simulink model "fourCars"  (R2024a)
settings: Solver=FixedStepAuto  StartTime=0.0  StopTime=config.t_max  FixedStep=config.timestep  RelTol=1e-3
undefined symbols (not defined in the file or in its folder): agentsInfo, config, DiscIntNeverNeededParam, Sim3dSensor
libraries: sim3dlib x6, dspvision x1, visionsinks x1
settings Model: Creator=alexs  LastModifiedBy=alexs

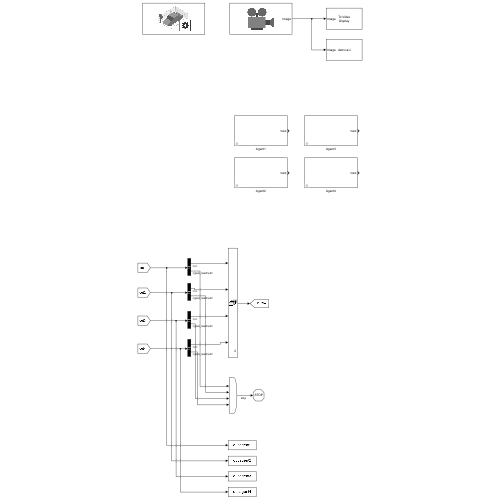
[thumbnail: Simulink's stored preview of the top-level diagram]
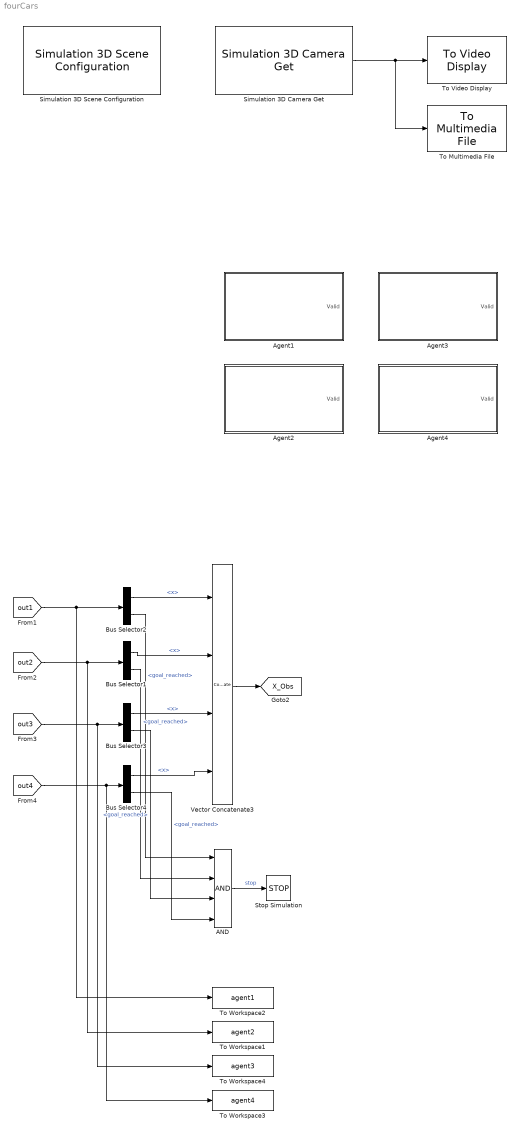
== system fourCars ==
  AND : Logic  Inputs=4  IconShape=distinctive  AllPortsSameDT=off  OutDataTypeStr=boolean
  Agent1 : Subsystem  mask{id=1, allAgentsInfo=agentsInfo}
      mask prompts: id "Identifier"; allAgentsInfo "Agents information"
  Agent2 : Subsystem  mask{id=2, allAgentsInfo=agentsInfo}
      mask prompts: id "Identifier"; allAgentsInfo "Agents information"
  Agent3 : Subsystem  mask{id=3, allAgentsInfo=agentsInfo}
      mask prompts: id "Identifier"; allAgentsInfo "Agents information"
  Agent4 : Subsystem  mask{id=4, allAgentsInfo=agentsInfo}
      mask prompts: id "Identifier"; allAgentsInfo "Agents information"
  Bus Selector{1..4} (4 alike) : BusSelector  OutputSignals=x,goal_reached
  Simulation 3D Camera Get : sim3dlib/Simulation 3D Camera Get  Priority=1  sensorTag=Sim3dSensor�  sensorId=1  sensorName=Sim3dSensor�  vehTagList={'Scene Origin';'actor1000'}  vehTag=Scene Origin  mountLoc=Origin  offsetFlag=on  tmountOffset=cameraTranslation  rmountOffset=cameraRotation  HorizontalResolution=1280  VerticalResolution=720  HorizontalFOV=60  SampleTime=-1  mountPoint=[0 0 40]  mountOrientation=[0 -90 -90]  aMode=5  ID=1
      settings: LibrarySourceBlock=sl3dlib/Simulation 3D/Utilities/Simulation 3D Camera Get
  Simulation 3D Scene Configuration : sim3dlib/Simulation 3D Scene Configuration  Priority=0  ProjectFormat=Default Scenes  SceneDesc=Empty scene  ProjectName=C:\Program Files\MATLAB\R2024a\toolbox\shared\sim3d_projects\automotive_project_windows\UE\WindowsNoEditor\VehicleSimulation.exe  ScenePath=/Game/Maps/HwStrght  EnableOpenDRIVE=off  vehTagList={'Custom';'Scene Origin';'actor1000'}  vehTag=Scene Origin  FreeCameraInitialTranslation=[0, 0, 0]  FreeCameraDefaultInitialTranslation=[-6, 0, 2]  FreeCameraInitialRotation=[0, 0, 0]  FreeCameraDefaultInitialRotation=[0, -15, 0]  OpVisEn=off  Ts=config.timestep  EnableWindow=off  EnableRemoteAccess=off  EnableWeather=off  SunAzimuth=90  SunAltitude=40.0  EnableGeospatialSun=off  Latitude=0  Longitude=0  Date=2023-01-01  Time=10:30:00  GeoTimeZone=-5.0  SunDaylightSaving=off  wind=1  clouds=10  EnableVolumetricClouds=off  CloudCoverage=0  CloudAltitude=6  fog=0  rain=0  RaindropsEffect=off  SnowDensity=0  EnableGeospatial=off  UseTrueOrigin=off  OriginHeight=200  OriginLatitude=40.744652  OriginLongitude=-73.988864  MapStyle=Aerial  AdditionalAssetIDs=[]  UseAdvancedSunSky=off  SolarTime=11  TimeZone=-5  Day=21  Month=9  Year=2022  UseDaylightSavingTime=on  DSTStartDay=10  DSTStartMonth=3  DSTEndDay=3  DSTEndMonth=11  DSTSwitchHour=2  sensorTag=MainCamera1  sensorId=1  sensorName=MainCamera1  mountLoc=Origin  offsetFlag=off  tmountOffset=[0, 0, 0]  rmountOffset=[0, 0, 0]  HorizontalResolution=1280  VerticalResolution=720  HorizontalFOV=60  mountPoint=[0 0 0]  mountOrientation=[0 0 0]  aMode=5  ID=1  GeoTrigger=Inactive
      settings: LibrarySourceBlock=sl3dlib/Simulation 3D/Environment/Simulation 3D Scene Configuration
  Stop Simulation : Stop
  To Multimedia File : dspvision/To Multimedia File  outputFilename=demo.avi  streamSelection=Video only  videoCompressor=None (uncompressed)  audioCompressor=None (uncompressed)  imagePorts=One multidimensional signal  fileType=AVI  audioDatatype=Determine from input data type  fourcc=RGB  audioBitRate=128  audioQuality=75  videoQuality=75  mj2000CompFactor=10
      settings: LibrarySourceBlock=visionsinks/To Multimedia File
  To Video Display : visionsinks/To Video Display  windowSizeMode=Normal  openAtMdlStart=on  fullScreen=off  videoWindowX=536805376  videoWindowY=536805376  saveWindowSize=off  videoWindowWidth=808  videoWindowHeight=639  inputColorFormat=RGB  inputType=Obsolete  imagePorts=One multidimensional signal  OutputDevice=On-screen video monitor  dataOrg=Column-major  isWindowOpen=off
  To Workspace1 : ToWorkspace  VariableName=agent2  SaveFormat=Timeseries  SampleTime=-1
  To Workspace2 : ToWorkspace  VariableName=agent1  SaveFormat=Timeseries  SampleTime=-1
  To Workspace3 : ToWorkspace  VariableName=agent4  SaveFormat=Timeseries  SampleTime=-1
  To Workspace4 : ToWorkspace  VariableName=agent3  SaveFormat=Timeseries  SampleTime=-1
  Vector Concatenate3 : Concatenate  NumInputs=4  Mode=Multidimensional array  ConcatenateDimension=2
  tag scope: X_Obs=global
  wires:
  Simulation 3D Camera Get/1 -> To Multimedia File/1, To Video Display/1
  [out1] -> To Workspace2/1, Bus Selector2/1
  Bus Selector2/1 -> Vector Concatenate3/1  "<x>"
  Vector Concatenate3/1 -> [X_Obs]
  Bus Selector2/2 -> AND/1  "<goal_reached>"
  AND/1 -> Stop Simulation/1  "stop"
  [out2] -> Bus Selector1/1, To Workspace1/1
  Bus Selector1/1 -> Vector Concatenate3/2  "<x>"
  Bus Selector1/2 -> AND/2  "<goal_reached>"
  [out3] -> To Workspace4/1, Bus Selector3/1
  [out4] -> To Workspace3/1, Bus Selector4/1
  Bus Selector3/1 -> Vector Concatenate3/3  "<x>"
  Bus Selector4/1 -> Vector Concatenate3/4  "<x>"
  Bus Selector3/2 -> AND/3  "<goal_reached>"
  Bus Selector4/2 -> AND/4  "<goal_reached>"

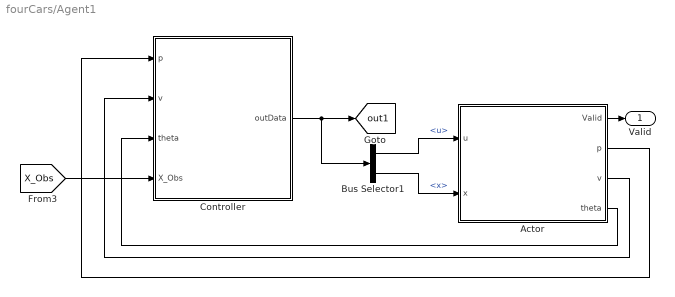
== system fourCars/Agent1 ==
  Actor : Subsystem
  Bus Selector1 : BusSelector  OutputSignals=u,x
  Controller : Subsystem  mask{id=id, allAgentsInfo=agentsInfo}
      mask prompts: id "Identifier"; allAgentsInfo "Information for all agents"
  Valid : Outport
  tag scope: out1=global
  wires:
  Actor/3(v) -> Controller/2(v)
  Controller/1(outData) -> Bus Selector1/1, [out1]
  Actor/2(p) -> Controller/1(p)
  Bus Selector1/1 -> Actor/1(u)  "<u>"
  [X_Obs] -> Controller/4(X_Obs)
  Actor/1(Valid) -> Valid/1
  Actor/4(theta) -> Controller/3(theta)
  Bus Selector1/2 -> Actor/2(x)  "<x>"

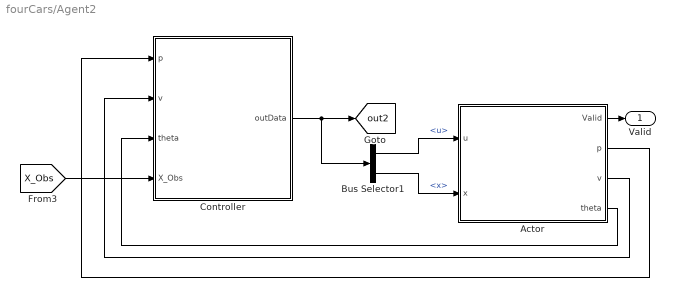
== system fourCars/Agent2 ==
  Actor : Subsystem
  Bus Selector1 : BusSelector  OutputSignals=u,x
  Controller : Subsystem  mask{id=id, allAgentsInfo=agentsInfo}
      mask prompts: id "Identifier"; allAgentsInfo "Information for all agents"
  Valid : Outport
  tag scope: out2=global
  wires:
  Bus Selector1/2 -> Actor/2(x)  "<x>"
  Actor/4(theta) -> Controller/3(theta)
  Actor/1(Valid) -> Valid/1
  [X_Obs] -> Controller/4(X_Obs)
  Bus Selector1/1 -> Actor/1(u)  "<u>"
  Actor/2(p) -> Controller/1(p)
  Controller/1(outData) -> [out2], Bus Selector1/1
  Actor/3(v) -> Controller/2(v)

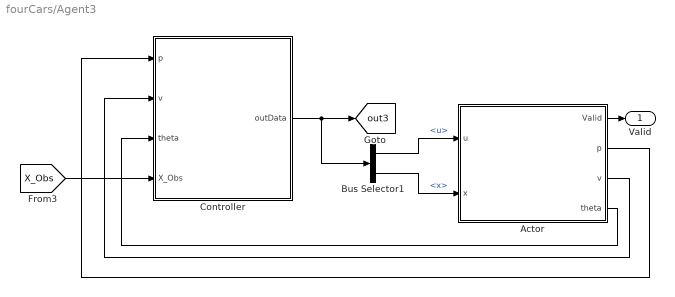
== system fourCars/Agent3 ==
  Actor : Subsystem
  Bus Selector1 : BusSelector  OutputSignals=u,x
  Controller : Subsystem  mask{id=id, allAgentsInfo=agentsInfo}
      mask prompts: id "Identifier"; allAgentsInfo "Information for all agents"
  Valid : Outport
  tag scope: out3=global
  wires:
  Bus Selector1/2 -> Actor/2(x)  "<x>"
  Actor/4(theta) -> Controller/3(theta)
  Actor/1(Valid) -> Valid/1
  [X_Obs] -> Controller/4(X_Obs)
  Bus Selector1/1 -> Actor/1(u)  "<u>"
  Actor/2(p) -> Controller/1(p)
  Controller/1(outData) -> [out3], Bus Selector1/1
  Actor/3(v) -> Controller/2(v)

== system fourCars/Agent4 ==
  Actor : Subsystem
  Bus Selector1 : BusSelector  OutputSignals=u,x
  Controller : Subsystem  mask{id=id, allAgentsInfo=agentsInfo}
      mask prompts: id "Identifier"; allAgentsInfo "Information for all agents"
  Valid : Outport
  tag scope: out4=global
  wires:
  Actor/3(v) -> Controller/2(v)
  Controller/1(outData) -> Bus Selector1/1, [out4]
  Actor/2(p) -> Controller/1(p)
  Bus Selector1/1 -> Actor/1(u)  "<u>"
  [X_Obs] -> Controller/4(X_Obs)
  Actor/1(Valid) -> Valid/1
  Actor/4(theta) -> Controller/3(theta)
  Bus Selector1/2 -> Actor/2(x)  "<x>"

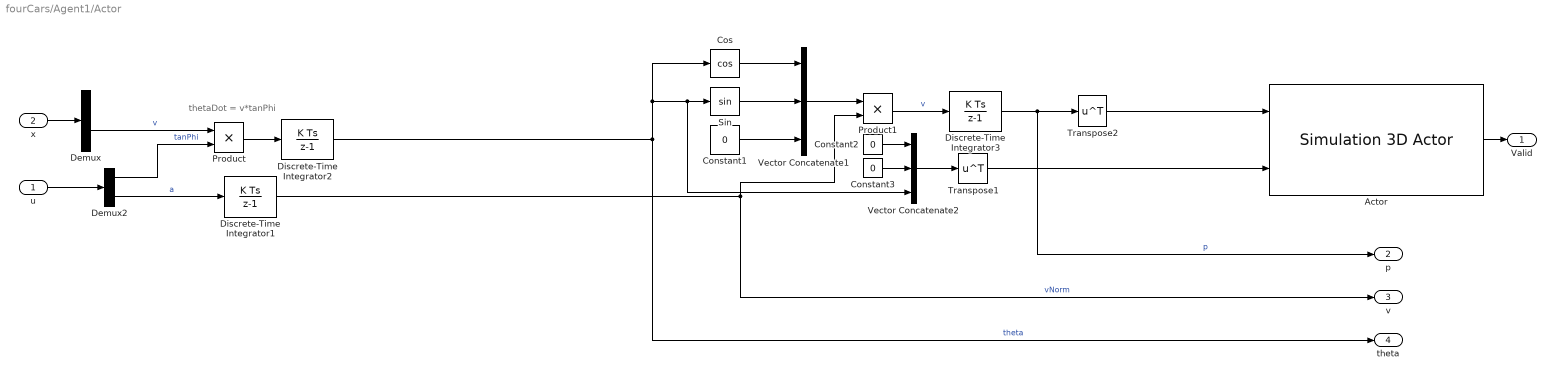
== system fourCars/Agent1/Actor ==
  note: thetaDot = v*tanPhi
  u : Inport
  x : Inport  Port=2
  Actor : sim3dlib/Simulation 3D Actor  Priority=1  ActorName=actor1  ParentName=Scene Origin  Operation=Create at setup  InitScriptText=|  SampleTime=-1  Translation=agentsInfo{id}.p'  Rotation=single([0 0 0])  Scale=single([1 1 1])  InputsText=actor1.Translation actor1.Rotation  aMode=5  ActorTag=actor1  ActorType=Sim3dActor  ID=C
      | % Reserved keywords:
      | % - Actor : handle to this actor object
      | % - World : handle to the world object
      | 
      | % Examples:
      | 
      | % Create a primitive geometry (optional)
      | 
      | % Actor.createShape('sphere', [allAgentsInfo{id}.shape(1) allAgentsInfo{id}.shape(2) 1]);
      | 
      | 
      | % Initialize values (optional)
      | % Actor.Scale = 1;
      | % Actor.Gravity = false;
      | % Actor.Physics = true;
      | % Actor.Color = [0 0 1];
      | % Actor.Shininess = 0;
      | % Actor.Mobility = sim3d.utils.MobilityTypes.Movable;
      | % Actor.Shadows = false;
  Constant1 : Constant  Value=0
  Constant2 : Constant  Value=0
  Constant3 : Constant  Value=0
  Cos : Trigonometry  Operator=cos
  Demux : Demux  Outputs=5
  Demux2 : Demux  Outputs=2
  Discrete-Time Integrator1 : DiscreteIntegrator  InitialCondition=agentsInfo{id}.v  SampleTime=-1  LimitOutput=on  UpperSaturationLimit=config.v_max/sqrt(2)  LowerSaturationLimit=-config.v_max/sqrt(2)  ICPrevOutput=DiscIntNeverNeededParam  ICPrevScaledInput=DiscIntNeverNeededParam
  Discrete-Time Integrator2 : DiscreteIntegrator  InitialCondition=agentsInfo{id}.theta  SampleTime=-1  ICPrevOutput=DiscIntNeverNeededParam  ICPrevScaledInput=DiscIntNeverNeededParam
  Discrete-Time Integrator3 : DiscreteIntegrator  InitialCondition=agentsInfo{id}.p  SampleTime=-1  UpperSaturationLimit=config.vMax  LowerSaturationLimit=-config.vMax  ICPrevOutput=DiscIntNeverNeededParam  ICPrevScaledInput=DiscIntNeverNeededParam
  Product : Product
  Product1 : Product
  Sin : Trigonometry
  Transpose1 : Math  Operator=transpose
  Transpose2 : Math  Operator=transpose
  Vector Concatenate1 : Concatenate  NumInputs=3
  Vector Concatenate2 : Concatenate  NumInputs=3
  Valid : Outport
  p : Outport  Port=2
  v : Outport  Port=3
  theta : Outport  Port=4
  wires:
  Actor/1 -> Valid/1
  Product/1 -> Discrete-Time Integrator2/1
  Demux2/1 -> Product/2  "tanPhi"
  Demux2/2 -> Discrete-Time Integrator1/1  "a"
  Discrete-Time Integrator2/1 -> Vector Concatenate2/3, Sin/1, Cos/1, theta/1  "theta"
  u/1 -> Demux2/1
  Discrete-Time Integrator1/1 -> Product1/2, v/1  "vNorm"
  Cos/1 -> Vector Concatenate1/1
  Sin/1 -> Vector Concatenate1/2
  Constant1/1 -> Vector Concatenate1/3
  Vector Concatenate1/1 -> Product1/1
  Product1/1 -> Discrete-Time Integrator3/1  "v"
  Discrete-Time Integrator3/1 -> p/1, Transpose2/1  "p"
  Transpose2/1 -> Actor/1
  x/1 -> Demux/1
  Demux/4 -> Product/1  "v"
  Constant2/1 -> Vector Concatenate2/1
  Constant3/1 -> Vector Concatenate2/2
  Vector Concatenate2/1 -> Transpose1/1
  Transpose1/1 -> Actor/2

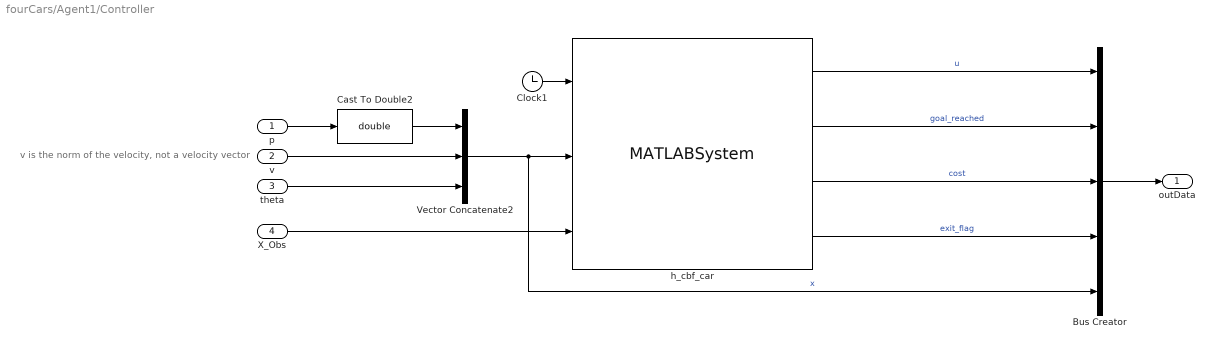
== system fourCars/Agent1/Controller ==
  note: v is the norm of the velocity, not a velocity vector
  p : Inport
  v : Inport  Port=2
  theta : Inport  Port=3
  X_Obs : Inport  Port=4
  Bus Creator : BusCreator  Inputs=5
  Cast To Double2 : DataTypeConversion  OutDataTypeStr=double  SaturateOnIntegerOverflow=off  RndMeth=Floor
  Clock1 : Clock
  Vector Concatenate2 : Concatenate  NumInputs=3
  h_cbf_car : MATLABSystem  System=h_cbf_car  id=id  config=config  agents_info=agentsInfo  SimulateUsing=Interpreted execution
      mask Type: h_cbf_car
      mask Display:
      | disp('h_cbf_car');
      | port_label('input',1,'t');
      | port_label('input',2,'x');
      | port_label('input',3,'X_obs');
      | port_label('output',1,'u');
      | port_label('output',2,'goal_reached');
      | port_label('output',3,'cost');
      | port_label('output',4,'exit_flag');
  outData : Outport
  wires:
  Vector Concatenate2/1 -> Bus Creator/5, h_cbf_car/2  "x"
  h_cbf_car/4 -> Bus Creator/4  "exit_flag"
  Bus Creator/1 -> outData/1
  Clock1/1 -> h_cbf_car/1
  h_cbf_car/3 -> Bus Creator/3  "cost"
  Cast To Double2/1 -> Vector Concatenate2/1
  h_cbf_car/1 -> Bus Creator/1  "u"
  p/1 -> Cast To Double2/1
  X_Obs/1 -> h_cbf_car/3
  h_cbf_car/2 -> Bus Creator/2  "goal_reached"
  v/1 -> Vector Concatenate2/2
  theta/1 -> Vector Concatenate2/3

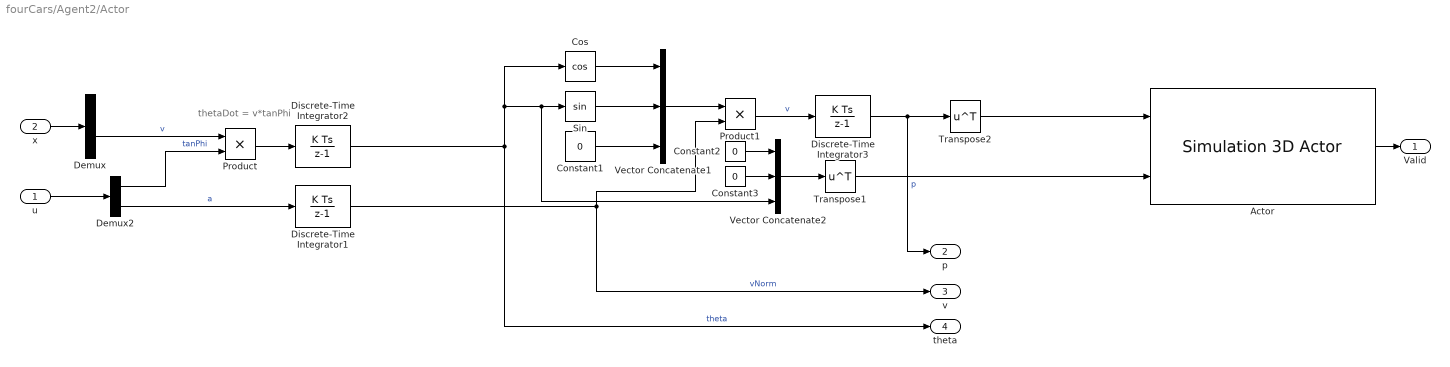
== system fourCars/Agent2/Actor ==
  note: thetaDot = v*tanPhi
  u : Inport
  x : Inport  Port=2
  Actor : sim3dlib/Simulation 3D Actor  Priority=1  ActorName=actor2  ParentName=Scene Origin  Operation=Create at setup  InitScriptText=|  SampleTime=-1  Translation=agentsInfo{id}.p'  Rotation=single([0 0 0])  Scale=single([1 1 1])  InputsText=actor2.Translation actor2.Rotation  aMode=5  ActorTag=actor2  ActorType=Sim3dActor  ID=C
      | % Reserved keywords:
      | % - Actor : handle to this actor object
      | % - World : handle to the world object
      | 
      | % Examples:
      | 
      | % Create a primitive geometry (optional)
      | 
      | % Actor.createShape('sphere', [allAgentsInfo{id}.shape(1) allAgentsInfo{id}.shape(2) 1]);
      | 
      | 
      | % Initialize values (optional)
      | % Actor.Scale = 1;
      | % Actor.Gravity = false;
      | % Actor.Physics = true;
      | % Actor.Color = [0 0 1];
      | % Actor.Shininess = 0;
      | % Actor.Mobility = sim3d.utils.MobilityTypes.Movable;
      | % Actor.Shadows = false;
  Constant1 : Constant  Value=0
  Constant2 : Constant  Value=0
  Constant3 : Constant  Value=0
  Cos : Trigonometry  Operator=cos
  Demux : Demux  Outputs=5
  Demux2 : Demux  Outputs=2
  Discrete-Time Integrator1 : DiscreteIntegrator  InitialCondition=agentsInfo{id}.v  SampleTime=-1  LimitOutput=on  UpperSaturationLimit=config.v_max/sqrt(2)  LowerSaturationLimit=-config.v_max/sqrt(2)  ICPrevOutput=DiscIntNeverNeededParam  ICPrevScaledInput=DiscIntNeverNeededParam
  Discrete-Time Integrator2 : DiscreteIntegrator  InitialCondition=agentsInfo{id}.theta  SampleTime=-1  ICPrevOutput=DiscIntNeverNeededParam  ICPrevScaledInput=DiscIntNeverNeededParam
  Discrete-Time Integrator3 : DiscreteIntegrator  InitialCondition=agentsInfo{id}.p  SampleTime=-1  UpperSaturationLimit=config.vMax  LowerSaturationLimit=-config.vMax  ICPrevOutput=DiscIntNeverNeededParam  ICPrevScaledInput=DiscIntNeverNeededParam
  Product : Product
  Product1 : Product
  Sin : Trigonometry
  Transpose1 : Math  Operator=transpose
  Transpose2 : Math  Operator=transpose
  Vector Concatenate1 : Concatenate  NumInputs=3
  Vector Concatenate2 : Concatenate  NumInputs=3
  Valid : Outport
  p : Outport  Port=2
  v : Outport  Port=3
  theta : Outport  Port=4
  wires:
  Transpose1/1 -> Actor/2
  Vector Concatenate2/1 -> Transpose1/1
  Constant3/1 -> Vector Concatenate2/2
  Constant2/1 -> Vector Concatenate2/1
  Demux/4 -> Product/1  "v"
  x/1 -> Demux/1
  Transpose2/1 -> Actor/1
  Discrete-Time Integrator3/1 -> Transpose2/1, p/1  "p"
  Product1/1 -> Discrete-Time Integrator3/1  "v"
  Vector Concatenate1/1 -> Product1/1
  Constant1/1 -> Vector Concatenate1/3
  Sin/1 -> Vector Concatenate1/2
  Cos/1 -> Vector Concatenate1/1
  Discrete-Time Integrator1/1 -> v/1, Product1/2  "vNorm"
  u/1 -> Demux2/1
  Discrete-Time Integrator2/1 -> theta/1, Cos/1, Sin/1, Vector Concatenate2/3  "theta"
  Demux2/2 -> Discrete-Time Integrator1/1  "a"
  Demux2/1 -> Product/2  "tanPhi"
  Product/1 -> Discrete-Time Integrator2/1
  Actor/1 -> Valid/1

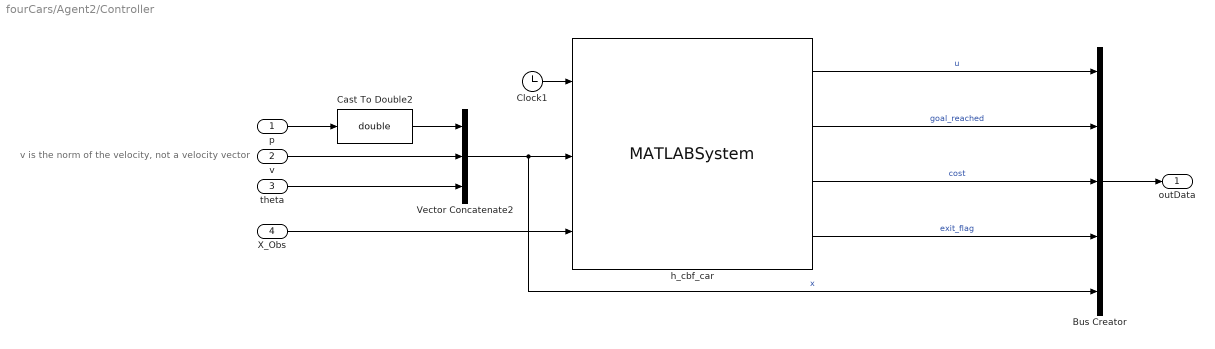
== system fourCars/Agent2/Controller ==
  note: v is the norm of the velocity, not a velocity vector
  p : Inport
  v : Inport  Port=2
  theta : Inport  Port=3
  X_Obs : Inport  Port=4
  Bus Creator : BusCreator  Inputs=5
  Cast To Double2 : DataTypeConversion  OutDataTypeStr=double  SaturateOnIntegerOverflow=off  RndMeth=Floor
  Clock1 : Clock
  Vector Concatenate2 : Concatenate  NumInputs=3
  h_cbf_car : MATLABSystem  System=h_cbf_car  id=id  config=config  agents_info=agentsInfo  SimulateUsing=Interpreted execution
      mask Type: h_cbf_car
      mask Display:
      | disp('h_cbf_car');
      | port_label('input',1,'t');
      | port_label('input',2,'x');
      | port_label('input',3,'X_obs');
      | port_label('output',1,'u');
      | port_label('output',2,'goal_reached');
      | port_label('output',3,'cost');
      | port_label('output',4,'exit_flag');
  outData : Outport
  wires:
  theta/1 -> Vector Concatenate2/3
  v/1 -> Vector Concatenate2/2
  h_cbf_car/2 -> Bus Creator/2  "goal_reached"
  X_Obs/1 -> h_cbf_car/3
  p/1 -> Cast To Double2/1
  h_cbf_car/1 -> Bus Creator/1  "u"
  Cast To Double2/1 -> Vector Concatenate2/1
  h_cbf_car/3 -> Bus Creator/3  "cost"
  Clock1/1 -> h_cbf_car/1
  Bus Creator/1 -> outData/1
  h_cbf_car/4 -> Bus Creator/4  "exit_flag"
  Vector Concatenate2/1 -> h_cbf_car/2, Bus Creator/5  "x"

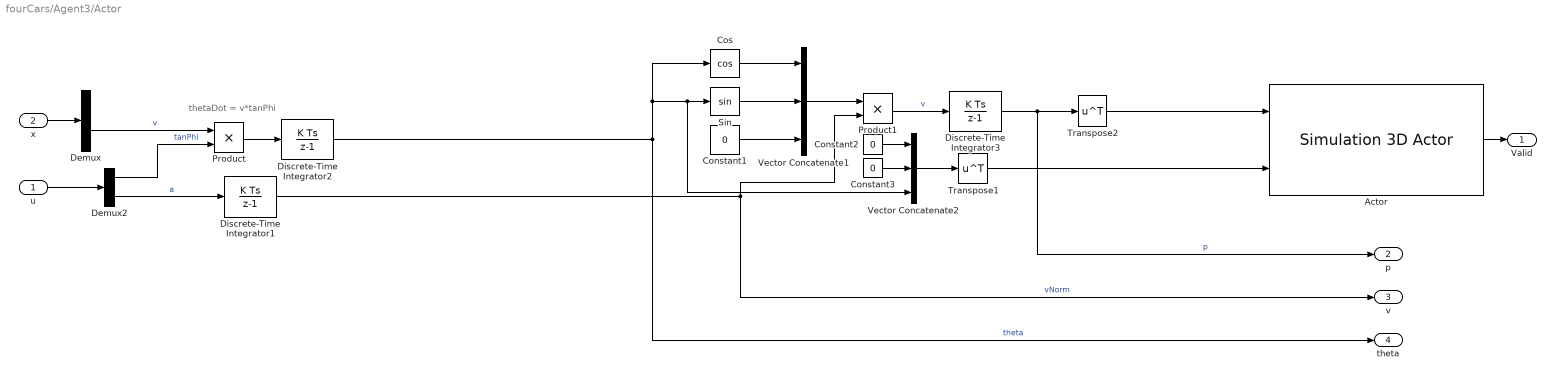
== system fourCars/Agent3/Actor ==
  note: thetaDot = v*tanPhi
  u : Inport
  x : Inport  Port=2
  Actor : sim3dlib/Simulation 3D Actor  Priority=1  ActorName=actor3  ParentName=Scene Origin  Operation=Create at setup  InitScriptText=|  SampleTime=-1  Translation=agentsInfo{id}.p'  Rotation=single([0 0 0])  Scale=single([1 1 1])  InputsText=actor3.Translation actor3.Rotation  aMode=5  ActorTag=actor3  ActorType=Sim3dActor  ID=C
      | % Reserved keywords:
      | % - Actor : handle to this actor object
      | % - World : handle to the world object
      | 
      | % Examples:
      | 
      | % Create a primitive geometry (optional)
      | 
      | % Actor.createShape('sphere', [allAgentsInfo{id}.shape(1) allAgentsInfo{id}.shape(2) 1]);
      | 
      | 
      | % Initialize values (optional)
      | % Actor.Scale = 1;
      | % Actor.Gravity = false;
      | % Actor.Physics = true;
      | % Actor.Color = [0 0 1];
      | % Actor.Shininess = 0;
      | % Actor.Mobility = sim3d.utils.MobilityTypes.Movable;
      | % Actor.Shadows = false;
  Constant1 : Constant  Value=0
  Constant2 : Constant  Value=0
  Constant3 : Constant  Value=0
  Cos : Trigonometry  Operator=cos
  Demux : Demux  Outputs=5
  Demux2 : Demux  Outputs=2
  Discrete-Time Integrator1 : DiscreteIntegrator  InitialCondition=agentsInfo{id}.v  SampleTime=-1  LimitOutput=on  UpperSaturationLimit=config.v_max/sqrt(2)  LowerSaturationLimit=-config.v_max/sqrt(2)  ICPrevOutput=DiscIntNeverNeededParam  ICPrevScaledInput=DiscIntNeverNeededParam
  Discrete-Time Integrator2 : DiscreteIntegrator  InitialCondition=agentsInfo{id}.theta  SampleTime=-1  ICPrevOutput=DiscIntNeverNeededParam  ICPrevScaledInput=DiscIntNeverNeededParam
  Discrete-Time Integrator3 : DiscreteIntegrator  InitialCondition=agentsInfo{id}.p  SampleTime=-1  UpperSaturationLimit=config.vMax  LowerSaturationLimit=-config.vMax  ICPrevOutput=DiscIntNeverNeededParam  ICPrevScaledInput=DiscIntNeverNeededParam
  Product : Product
  Product1 : Product
  Sin : Trigonometry
  Transpose1 : Math  Operator=transpose
  Transpose2 : Math  Operator=transpose
  Vector Concatenate1 : Concatenate  NumInputs=3
  Vector Concatenate2 : Concatenate  NumInputs=3
  Valid : Outport
  p : Outport  Port=2
  v : Outport  Port=3
  theta : Outport  Port=4
  wires:
  Transpose1/1 -> Actor/2
  Vector Concatenate2/1 -> Transpose1/1
  Constant3/1 -> Vector Concatenate2/2
  Constant2/1 -> Vector Concatenate2/1
  Demux/4 -> Product/1  "v"
  x/1 -> Demux/1
  Transpose2/1 -> Actor/1
  Discrete-Time Integrator3/1 -> Transpose2/1, p/1  "p"
  Product1/1 -> Discrete-Time Integrator3/1  "v"
  Vector Concatenate1/1 -> Product1/1
  Constant1/1 -> Vector Concatenate1/3
  Sin/1 -> Vector Concatenate1/2
  Cos/1 -> Vector Concatenate1/1
  Discrete-Time Integrator1/1 -> v/1, Product1/2  "vNorm"
  u/1 -> Demux2/1
  Discrete-Time Integrator2/1 -> theta/1, Cos/1, Sin/1, Vector Concatenate2/3  "theta"
  Demux2/2 -> Discrete-Time Integrator1/1  "a"
  Demux2/1 -> Product/2  "tanPhi"
  Product/1 -> Discrete-Time Integrator2/1
  Actor/1 -> Valid/1

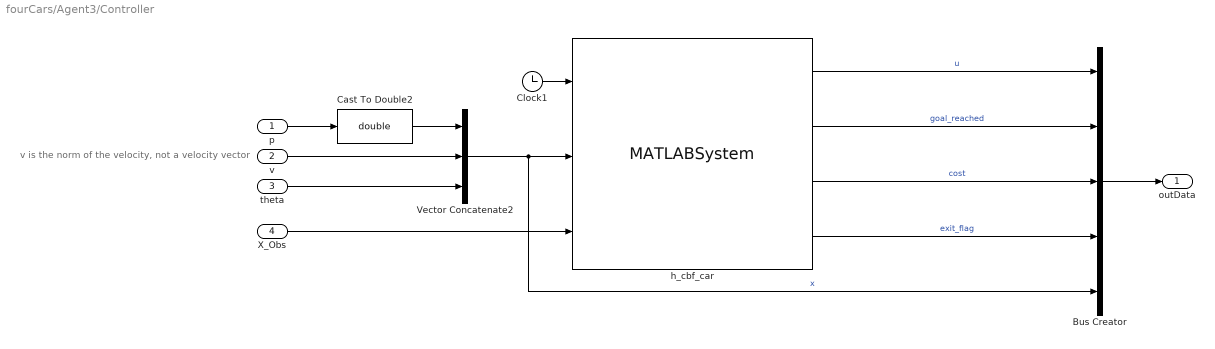
== system fourCars/Agent3/Controller ==
  note: v is the norm of the velocity, not a velocity vector
  p : Inport
  v : Inport  Port=2
  theta : Inport  Port=3
  X_Obs : Inport  Port=4
  Bus Creator : BusCreator  Inputs=5
  Cast To Double2 : DataTypeConversion  OutDataTypeStr=double  SaturateOnIntegerOverflow=off  RndMeth=Floor
  Clock1 : Clock
  Vector Concatenate2 : Concatenate  NumInputs=3
  h_cbf_car : MATLABSystem  System=h_cbf_car  id=id  config=config  agents_info=agentsInfo  SimulateUsing=Interpreted execution
      mask Type: h_cbf_car
      mask Display:
      | disp('h_cbf_car');
      | port_label('input',1,'t');
      | port_label('input',2,'x');
      | port_label('input',3,'X_obs');
      | port_label('output',1,'u');
      | port_label('output',2,'goal_reached');
      | port_label('output',3,'cost');
      | port_label('output',4,'exit_flag');
  outData : Outport
  wires:
  theta/1 -> Vector Concatenate2/3
  v/1 -> Vector Concatenate2/2
  h_cbf_car/2 -> Bus Creator/2  "goal_reached"
  X_Obs/1 -> h_cbf_car/3
  p/1 -> Cast To Double2/1
  h_cbf_car/1 -> Bus Creator/1  "u"
  Cast To Double2/1 -> Vector Concatenate2/1
  h_cbf_car/3 -> Bus Creator/3  "cost"
  Clock1/1 -> h_cbf_car/1
  Bus Creator/1 -> outData/1
  h_cbf_car/4 -> Bus Creator/4  "exit_flag"
  Vector Concatenate2/1 -> h_cbf_car/2, Bus Creator/5  "x"

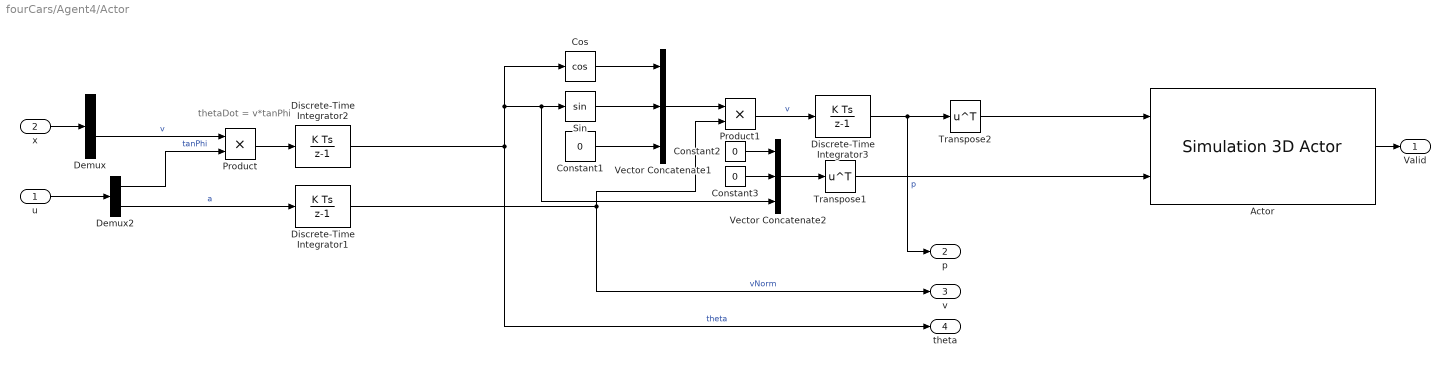
== system fourCars/Agent4/Actor ==
  note: thetaDot = v*tanPhi
  u : Inport
  x : Inport  Port=2
  Actor : sim3dlib/Simulation 3D Actor  Priority=1  ActorName=actor4  ParentName=Scene Origin  Operation=Create at setup  InitScriptText=|  SampleTime=-1  Translation=agentsInfo{id}.p'  Rotation=single([0 0 0])  Scale=single([1 1 1])  InputsText=actor4.Translation actor4.Rotation  aMode=5  ActorTag=actor4  ActorType=Sim3dActor  ID=C
      | % Reserved keywords:
      | % - Actor : handle to this actor object
      | % - World : handle to the world object
      | 
      | % Examples:
      | 
      | % Create a primitive geometry (optional)
      | 
      | % Actor.createShape('sphere', [allAgentsInfo{id}.shape(1) allAgentsInfo{id}.shape(2) 1]);
      | 
      | 
      | % Initialize values (optional)
      | % Actor.Scale = 1;
      | % Actor.Gravity = false;
      | % Actor.Physics = true;
      | % Actor.Color = [0 0 1];
      | % Actor.Shininess = 0;
      | % Actor.Mobility = sim3d.utils.MobilityTypes.Movable;
      | % Actor.Shadows = false;
  Constant1 : Constant  Value=0
  Constant2 : Constant  Value=0
  Constant3 : Constant  Value=0
  Cos : Trigonometry  Operator=cos
  Demux : Demux  Outputs=5
  Demux2 : Demux  Outputs=2
  Discrete-Time Integrator1 : DiscreteIntegrator  InitialCondition=agentsInfo{id}.v  SampleTime=-1  LimitOutput=on  UpperSaturationLimit=config.v_max/sqrt(2)  LowerSaturationLimit=-config.v_max/sqrt(2)  ICPrevOutput=DiscIntNeverNeededParam  ICPrevScaledInput=DiscIntNeverNeededParam
  Discrete-Time Integrator2 : DiscreteIntegrator  InitialCondition=agentsInfo{id}.theta  SampleTime=-1  ICPrevOutput=DiscIntNeverNeededParam  ICPrevScaledInput=DiscIntNeverNeededParam
  Discrete-Time Integrator3 : DiscreteIntegrator  InitialCondition=agentsInfo{id}.p  SampleTime=-1  UpperSaturationLimit=config.vMax  LowerSaturationLimit=-config.vMax  ICPrevOutput=DiscIntNeverNeededParam  ICPrevScaledInput=DiscIntNeverNeededParam
  Product : Product
  Product1 : Product
  Sin : Trigonometry
  Transpose1 : Math  Operator=transpose
  Transpose2 : Math  Operator=transpose
  Vector Concatenate1 : Concatenate  NumInputs=3
  Vector Concatenate2 : Concatenate  NumInputs=3
  Valid : Outport
  p : Outport  Port=2
  v : Outport  Port=3
  theta : Outport  Port=4
  wires:
  Actor/1 -> Valid/1
  Product/1 -> Discrete-Time Integrator2/1
  Demux2/1 -> Product/2  "tanPhi"
  Demux2/2 -> Discrete-Time Integrator1/1  "a"
  Discrete-Time Integrator2/1 -> Vector Concatenate2/3, Sin/1, Cos/1, theta/1  "theta"
  u/1 -> Demux2/1
  Discrete-Time Integrator1/1 -> Product1/2, v/1  "vNorm"
  Cos/1 -> Vector Concatenate1/1
  Sin/1 -> Vector Concatenate1/2
  Constant1/1 -> Vector Concatenate1/3
  Vector Concatenate1/1 -> Product1/1
  Product1/1 -> Discrete-Time Integrator3/1  "v"
  Discrete-Time Integrator3/1 -> p/1, Transpose2/1  "p"
  Transpose2/1 -> Actor/1
  x/1 -> Demux/1
  Demux/4 -> Product/1  "v"
  Constant2/1 -> Vector Concatenate2/1
  Constant3/1 -> Vector Concatenate2/2
  Vector Concatenate2/1 -> Transpose1/1
  Transpose1/1 -> Actor/2

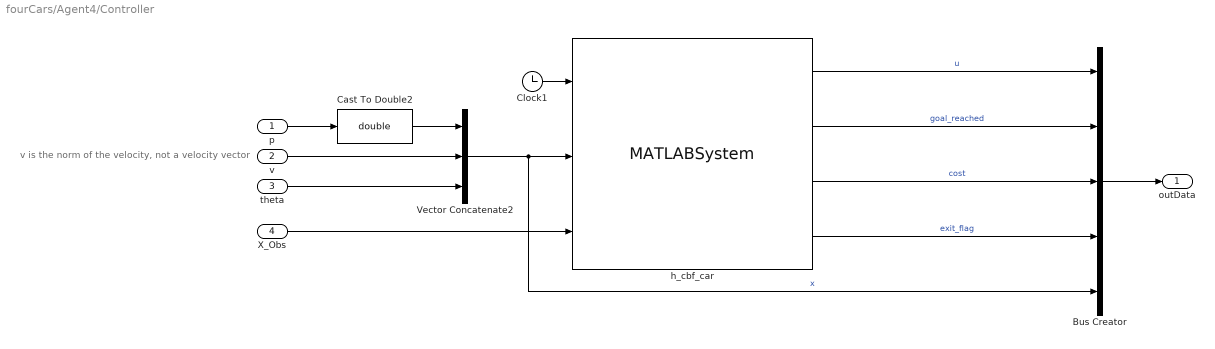
== system fourCars/Agent4/Controller ==
  note: v is the norm of the velocity, not a velocity vector
  p : Inport
  v : Inport  Port=2
  theta : Inport  Port=3
  X_Obs : Inport  Port=4
  Bus Creator : BusCreator  Inputs=5
  Cast To Double2 : DataTypeConversion  OutDataTypeStr=double  SaturateOnIntegerOverflow=off  RndMeth=Floor
  Clock1 : Clock
  Vector Concatenate2 : Concatenate  NumInputs=3
  h_cbf_car : MATLABSystem  System=h_cbf_car  id=id  config=config  agents_info=agentsInfo  SimulateUsing=Interpreted execution
      mask Type: h_cbf_car
      mask Display:
      | disp('h_cbf_car');
      | port_label('input',1,'t');
      | port_label('input',2,'x');
      | port_label('input',3,'X_obs');
      | port_label('output',1,'u');
      | port_label('output',2,'goal_reached');
      | port_label('output',3,'cost');
      | port_label('output',4,'exit_flag');
  outData : Outport
  wires:
  Vector Concatenate2/1 -> Bus Creator/5, h_cbf_car/2  "x"
  h_cbf_car/4 -> Bus Creator/4  "exit_flag"
  Bus Creator/1 -> outData/1
  Clock1/1 -> h_cbf_car/1
  h_cbf_car/3 -> Bus Creator/3  "cost"
  Cast To Double2/1 -> Vector Concatenate2/1
  h_cbf_car/1 -> Bus Creator/1  "u"
  p/1 -> Cast To Double2/1
  X_Obs/1 -> h_cbf_car/3
  h_cbf_car/2 -> Bus Creator/2  "goal_reached"
  v/1 -> Vector Concatenate2/2
  theta/1 -> Vector Concatenate2/3
